simulink model "Mophong_Daodong_1phan2"  (R2021b)
settings: Solver=VariableStepAuto  StartTime=0.0  StopTime=5  RelTol=1e-3
undefined symbols (not defined in the file): a, b, cL1, cL2, cT1, cT2, Iy, kL1, kL2, kT1, kT2, M, m1, m2, q0, v
settings Model: Creator=jackl  LastModifiedBy=jackl

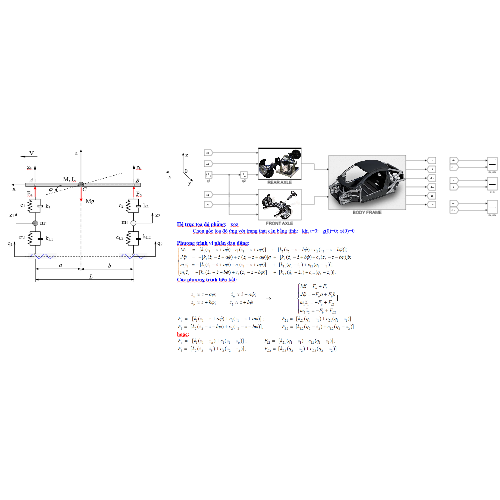
[thumbnail: Simulink's stored preview of the top-level diagram]
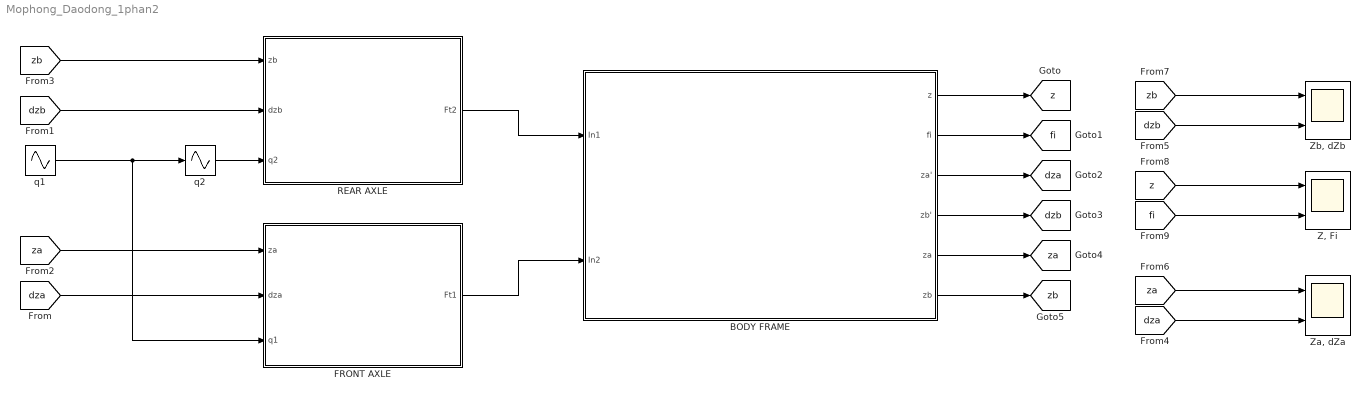
== system Mophong_Daodong_1phan2 ==
  BODY FRAME : Subsystem
      mask Display: image('D:\UDMT\Picture\Body.png'); % Use "Edit Image" on toolstrip to change.
  FRONT AXLE : Subsystem
      mask Display: image('D:\UDMT\Picture\cauTruoc.jpg'); % Use "Edit Image" on toolstrip to change.
  REAR AXLE : Subsystem
      mask Display: image('D:\UDMT\Picture\cauSau.jpg'); % Use "Edit Image" on toolstrip to change.
  "Z, Fi" : Scope  NumInputPorts=2
  "Za, dZa" : Scope  NumInputPorts=2
  "Zb, dZb" : Scope  NumInputPorts=2
  q1 : Sin  Amplitude=q0  Frequency=v  SampleTime=0
  q2 : Sin  TimeSource=Use external signal  SampleTime=0
  tag scope: dza=global, dzb=global, fi=global, z=global, za=global, zb=global
  wires:
  REAR AXLE/1(Ft2) -> BODY FRAME/1(In1)
  FRONT AXLE/1(Ft1) -> BODY FRAME/2(In2)
  BODY FRAME/1(z) -> [z]
  BODY FRAME/6(zb) -> [zb]
  BODY FRAME/2(fi) -> [fi]
  BODY FRAME/3(za') -> [dza]
  BODY FRAME/4(zb') -> [dzb]
  BODY FRAME/5(za) -> [za]
  [dza] -> FRONT AXLE/2(dza)
  [dzb] -> REAR AXLE/2(dzb)
  [za] -> FRONT AXLE/1(za)
  [zb] -> REAR AXLE/1(zb)
  q1/1 -> q2/1, FRONT AXLE/3(q1)
  q2/1 -> REAR AXLE/3(q2)
  [za] -> "Za, dZa"/1
  [dzb] -> "Zb, dZb"/2
  [dza] -> "Za, dZa"/2
  [zb] -> "Zb, dZb"/1
  [z] -> "Z, Fi"/1
  [fi] -> "Z, Fi"/2

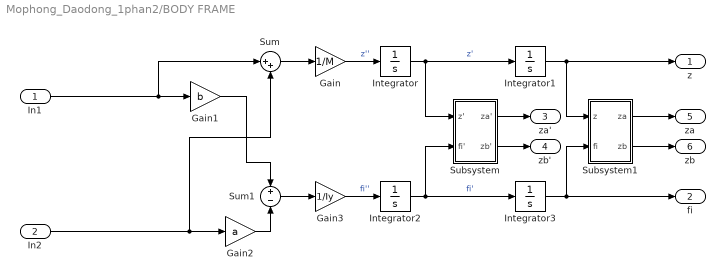
== system Mophong_Daodong_1phan2/BODY FRAME ==
  In1 : Inport
  In2 : Inport  Port=2
  Gain : Gain  Gain=1/M
  Gain1 : Gain  Gain=b
  Gain2 : Gain  Gain=a
  Gain3 : Gain  Gain=1/Iy
  Integrator{,1..3} (4 alike) : Integrator
  Subsystem : Subsystem
  Subsystem1 : Subsystem
  Sum : Sum  Inputs=|++
  Sum1 : Sum  Inputs=+-
  z : Outport
  fi : Outport  Port=2
  za' : Outport  Port=3
  zb' : Outport  Port=4
  za : Outport  Port=5
  zb : Outport  Port=6
  wires:
  Gain/1 -> Integrator/1  "z''"
  In1/1 -> Gain1/1, Sum/1
  In2/1 -> Gain2/1, Sum/2
  Subsystem/1(za') -> za'/1
  Sum/1 -> Gain/1
  Gain2/1 -> Sum1/2
  Subsystem1/1(za) -> za/1
  Subsystem1/2(zb) -> zb/1
  Integrator1/1 -> z/1, Subsystem1/1(z)
  Integrator2/1 -> Subsystem/2(fi'), Integrator3/1  "fi'"
  Subsystem/2(zb') -> zb'/1
  Sum1/1 -> Gain3/1
  Gain1/1 -> Sum1/1
  Integrator/1 -> Subsystem/1(z'), Integrator1/1  "z'"
  Integrator3/1 -> fi/1, Subsystem1/2(fi)
  Gain3/1 -> Integrator2/1  "fi''"

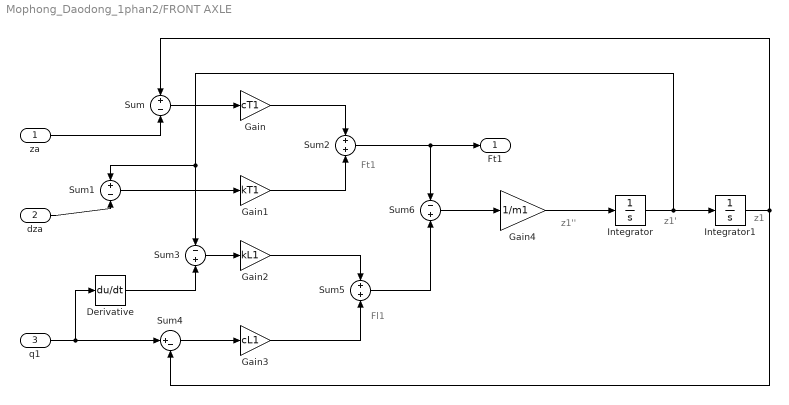
== system Mophong_Daodong_1phan2/FRONT AXLE ==
  note: z1
  note: z1'
  note: z1''
  note: Fl1
  note: Ft1
  za : Inport
  dza : Inport  Port=2
  q1 : Inport  Port=3
  Derivative : Derivative
  Gain : Gain  Gain=cT1
  Gain1 : Gain  Gain=kT1
  Gain2 : Gain  Gain=kL1
  Gain3 : Gain  Gain=cL1
  Gain4 : Gain  Gain=1/m1
  Integrator : Integrator
  Integrator1 : Integrator
  Sum : Sum  Inputs=+-
  Sum1 : Sum  Inputs=+-
  Sum2 : Sum
  Sum3 : Sum  Inputs=-+
  Sum4 : Sum  Inputs=|+-
  Sum5 : Sum
  Sum6 : Sum  Inputs=-+
  Ft1 : Outport
  wires:
  Sum/1 -> Gain/1
  dza/1 -> Sum1/2
  Sum3/1 -> Gain2/1
  Integrator/1 -> Sum1/1, Sum3/1, Integrator1/1
  q1/1 -> Sum4/1, Derivative/1
  Sum5/1 -> Sum6/2
  Sum4/1 -> Gain3/1
  Gain1/1 -> Sum2/2
  Sum2/1 -> Sum6/1, Ft1/1
  Integrator1/1 -> Sum4/2, Sum/1
  Gain4/1 -> Integrator/1
  Sum6/1 -> Gain4/1
  za/1 -> Sum/2
  Derivative/1 -> Sum3/2
  Sum1/1 -> Gain1/1
  Gain3/1 -> Sum5/2
  Gain2/1 -> Sum5/1
  Gain/1 -> Sum2/1

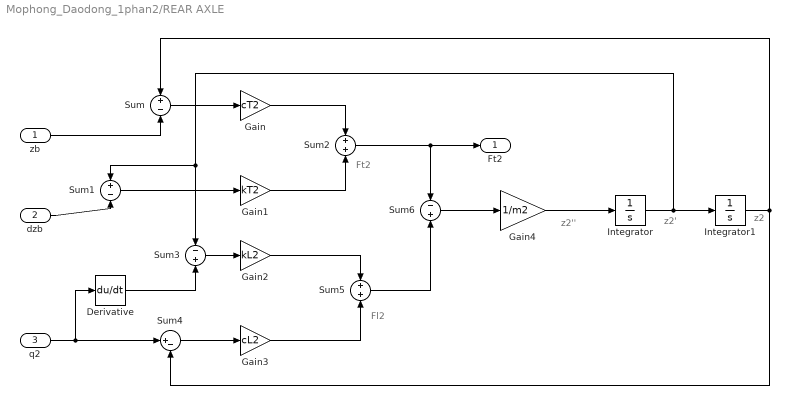
== system Mophong_Daodong_1phan2/REAR AXLE ==
  note: z2
  note: z2'
  note: z2''
  note: Fl2
  note: Ft2
  zb : Inport
  dzb : Inport  Port=2
  q2 : Inport  Port=3
  Derivative : Derivative
  Gain : Gain  Gain=cT2
  Gain1 : Gain  Gain=kT2
  Gain2 : Gain  Gain=kL2
  Gain3 : Gain  Gain=cL2
  Gain4 : Gain  Gain=1/m2
  Integrator : Integrator
  Integrator1 : Integrator
  Sum : Sum  Inputs=+-
  Sum1 : Sum  Inputs=+-
  Sum2 : Sum
  Sum3 : Sum  Inputs=-+
  Sum4 : Sum  Inputs=|+-
  Sum5 : Sum
  Sum6 : Sum  Inputs=-+
  Ft2 : Outport
  wires:
  Sum/1 -> Gain/1
  dzb/1 -> Sum1/2
  Sum3/1 -> Gain2/1
  Integrator/1 -> Sum1/1, Sum3/1, Integrator1/1
  q2/1 -> Sum4/1, Derivative/1
  Sum5/1 -> Sum6/2
  Sum4/1 -> Gain3/1
  Gain1/1 -> Sum2/2
  Sum2/1 -> Sum6/1, Ft2/1
  Integrator1/1 -> Sum4/2, Sum/1
  Gain4/1 -> Integrator/1
  Sum6/1 -> Gain4/1
  zb/1 -> Sum/2
  Derivative/1 -> Sum3/2
  Sum1/1 -> Gain1/1
  Gain3/1 -> Sum5/2
  Gain2/1 -> Sum5/1
  Gain/1 -> Sum2/1

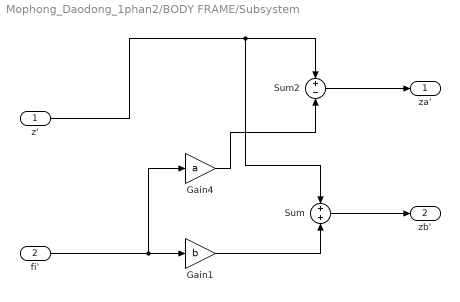
== system Mophong_Daodong_1phan2/BODY FRAME/Subsystem ==
  z' : Inport
  fi' : Inport  Port=2
  Gain1 : Gain  Gain=b
  Gain4 : Gain  Gain=a
  Sum : Sum
  Sum2 : Sum  Inputs=+-
  za' : Outport
  zb' : Outport  Port=2
  wires:
  fi'/1 -> Gain1/1, Gain4/1
  Gain4/1 -> Sum2/2
  Sum2/1 -> za'/1
  z'/1 -> Sum/1, Sum2/1
  Gain1/1 -> Sum/2
  Sum/1 -> zb'/1

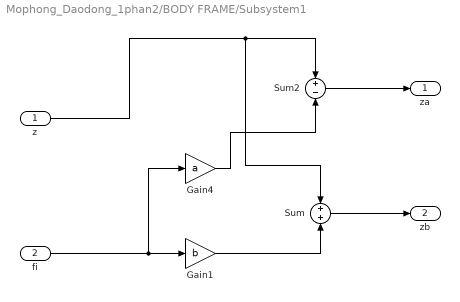
== system Mophong_Daodong_1phan2/BODY FRAME/Subsystem1 ==
  z : Inport
  fi : Inport  Port=2
  Gain1 : Gain  Gain=b
  Gain4 : Gain  Gain=a
  Sum : Sum
  Sum2 : Sum  Inputs=+-
  za : Outport
  zb : Outport  Port=2
  wires:
  fi/1 -> Gain1/1, Gain4/1
  Gain4/1 -> Sum2/2
  Sum2/1 -> za/1
  z/1 -> Sum/1, Sum2/1
  Gain1/1 -> Sum/2
  Sum/1 -> zb/1
